simulink model "surgicalControl_Shared_memory_loop_2016b"  (R2016b)
settings: Solver=FixedStepAuto  StartTime=0.0  StopTime=inf  FixedStep=1/100  RelTol=1e-3
libraries: dspsigops x9, simulink x3, matlabGenericSHM_Block x1
settings Model: Creator=daniel  LastModifiedBy=crazy
settings OptimizationCC: LifeSpan=inf
settings DebuggingCC: SFExecutionAtInitializationDiag=none

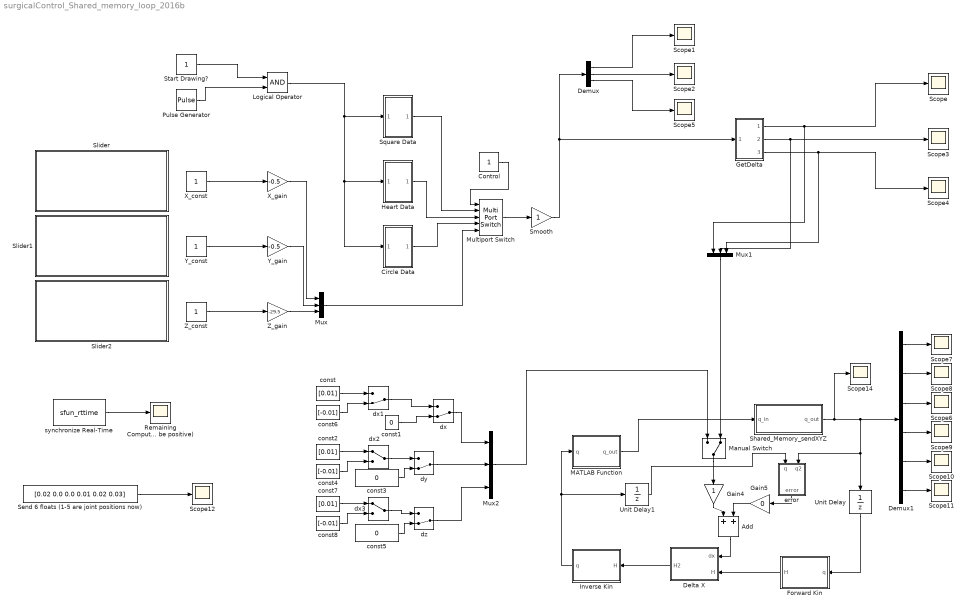
== system surgicalControl_Shared_memory_loop_2016b ==
  " GetDelta " : Subsystem
  " X_const " : Constant
  " Y_const" : Constant
  " Z_const" : Constant
  Add : Sum
  Circle Data : Subsystem
  "Control " : Constant
  Delta X : MATLAB Function  TreatAsAtomicUnit=on
  Demux : Demux  Outputs=3
  Demux1 : Demux  Outputs=6
  Forward Kin : MATLAB Function  TreatAsAtomicUnit=on
  Gain4 : Gain
  Gain5 : Gain  Gain=0
  Heart Data : Subsystem
  Inverse Kin : MATLAB Function  TreatAsAtomicUnit=on
  Logical Operator : Logic  AllPortsSameDT=off  OutDataTypeStr=boolean
  MATLAB Function : MATLAB Function  TreatAsAtomicUnit=on
  Manual Switch : ManualSwitch  CurrentSetting=0
  Multiport Switch : MultiPortSwitch  Inputs=4
  Mux : Mux  Inputs=3
  Mux1 : Mux  Inputs=3
  Mux2 : Mux  Inputs=3
  Pulse Generator : DiscretePulseGenerator  PulseType=Time based  Period=1  PulseWidth=20
  Remaining Computation Time (must be positive) : Scope
  Scope{,1..12,14} (14 alike) : Scope
  Send 6 floats (1-5 are joint positions now) : Constant  Value=[0.02 0.0 0.0 0.01 0.02 0.03]  OutDataTypeStr=single
  Shared_Memory_sendXYZ : Subsystem  mask{ID1=4}
  Slider : Subsystem  DialogController=hmiCreateDDGDialog  IsWebBlock=on  mask(MWDashboardBlock){webBlockId=4f94596f-dd6d-4e5e-bddc-7a8d913927f9, webBlockType=slider, ShowInLibBrowser=on, ShowInitialText=on, HMISrcModelName=surgicalControl_Shared_memory_loop_2016b}
      mask prompts: webBlockId "WebBlock Id"; webBlockType "WebBlock Type"; HMISrcModelName "Source Model"
      mask help: SimulinkHMI:dialogs:SliderDialogDesc
      mask Help: helpview([docroot '/mapfiles/simulink.map'], 'hmi_slider')
      mask Display:
      | if strcmp(get_param(bdroot(gcb),'BlockDiagramType'), 'library')
      |     image([(matlabroot) '/toolbox/simulink/hmi/icons/Slider.png']);
      | end
  Slider1 : Subsystem  DialogController=hmiCreateDDGDialog  IsWebBlock=on  mask(MWDashboardBlock){webBlockId=8aa996ad-7cd4-40fc-9a04-6a85939aea5d, webBlockType=slider, ShowInLibBrowser=on, ShowInitialText=on, HMISrcModelName=surgicalControl_Shared_memory_loop_2016b}
      mask prompts: webBlockId "WebBlock Id"; webBlockType "WebBlock Type"; HMISrcModelName "Source Model"
      mask help: SimulinkHMI:dialogs:SliderDialogDesc
      mask Help: helpview([docroot '/mapfiles/simulink.map'], 'hmi_slider')
      mask Display:
      | if strcmp(get_param(bdroot(gcb),'BlockDiagramType'), 'library')
      |     image([(matlabroot) '/toolbox/simulink/hmi/icons/Slider.png']);
      | end
  Slider2 : Subsystem  DialogController=hmiCreateDDGDialog  IsWebBlock=on  mask(MWDashboardBlock){webBlockId=1ddf6fd9-0225-4881-82ca-a25e179e2ab9, webBlockType=slider, ShowInLibBrowser=on, ShowInitialText=on, HMISrcModelName=surgicalControl_Shared_memory_loop_2016b}
      mask prompts: webBlockId "WebBlock Id"; webBlockType "WebBlock Type"; HMISrcModelName "Source Model"
      mask help: SimulinkHMI:dialogs:SliderDialogDesc
      mask Help: helpview([docroot '/mapfiles/simulink.map'], 'hmi_slider')
      mask Display:
      | if strcmp(get_param(bdroot(gcb),'BlockDiagramType'), 'library')
      |     image([(matlabroot) '/toolbox/simulink/hmi/icons/Slider.png']);
      | end
  Smooth : Gain
  "Square Data " : Subsystem
  Start Drawing? : Constant  SampleTime=1
  Unit Delay : UnitDelay  SampleTime=-1
  Unit Delay1 : UnitDelay  SampleTime=-1
  "X_gain " : Gain  Gain=-0.5
  "Y_gain " : Gain  Gain=-0.5
  Z_gain : Gain  Gain=-29.5
  const : Constant  Value=[0.01]  OutDataTypeStr=single
  const1 : Constant  Value=0  OutDataTypeStr=single
  const2 : Constant  Value=[0.01]  OutDataTypeStr=single
  const3 : Constant  Value=0  OutDataTypeStr=single
  const4 : Constant  Value=[-0.01]  OutDataTypeStr=single
  const5 : Constant  Value=0  OutDataTypeStr=single
  const6 : Constant  Value=[-0.01]  OutDataTypeStr=single
  const7 : Constant  Value=[0.01]  OutDataTypeStr=single
  const8 : Constant  Value=[-0.01]  OutDataTypeStr=single
  dx : ManualSwitch  CurrentSetting=0
  dx1 : ManualSwitch  CurrentSetting=0
  dx2 : ManualSwitch
  dx3 : ManualSwitch
  dy : ManualSwitch  CurrentSetting=0
  dz : ManualSwitch  CurrentSetting=0
  error : MATLAB Function  TreatAsAtomicUnit=on
  synchronize Real-Time : S-Function  FunctionName=sfun_rttime  Parameters=1  SFunctionDeploymentMode=off  EnableBusSupport=off
  wires:
  " GetDelta "/1(Out1) -> Mux1/1, Scope/1
  " GetDelta "/2(Out2) -> Scope3/1, Mux1/2
  " GetDelta "/3(Out3) -> Scope4/1, Mux1/3
  Multiport Switch/1 -> Smooth/1
  "Square Data "/1(xyz) -> Multiport Switch/2
  "Control "/1 -> Multiport Switch/1
  " X_const "/1 -> "X_gain "/1
  " Y_const"/1 -> "Y_gain "/1
  " Z_const"/1 -> Z_gain/1
  "X_gain "/1 -> Mux/1
  "Y_gain "/1 -> Mux/2
  Z_gain/1 -> Mux/3
  Mux/1 -> Multiport Switch/5
  Demux/2 -> Scope2/1
  Demux/1 -> Scope1/1
  Demux/3 -> Scope5/1
  synchronize Real-Time/1 -> Remaining Computation Time (must be positive)/1
  Smooth/1 -> Demux/1, " GetDelta "/1(In1)
  Shared_Memory_sendXYZ/1(q_out) -> Scope14/1, error/2(q2), Unit Delay/1, Demux1/1
  Demux1/3 -> Scope6/1
  Demux1/1 -> Scope7/1
  Demux1/2 -> Scope8/1
  Demux1/4 -> Scope9/1
  Demux1/5 -> Scope10/1
  Demux1/6 -> Scope11/1
  Send 6 floats (1-5 are joint positions now)/1 -> Scope12/1
  Forward Kin/1(H) -> Delta X/2(H)
  Delta X/1(H2) -> Inverse Kin/1(H)
  Unit Delay/1 -> Forward Kin/1(q)
  Mux1/1 -> Manual Switch/2
  Add/1 -> Delta X/1(dx)
  Mux2/1 -> Manual Switch/1
  dx/1 -> Mux2/1
  dx2/1 -> dy/1
  dy/1 -> Mux2/2
  dx3/1 -> dz/1
  dz/1 -> Mux2/3
  const/1 -> dx1/1
  const6/1 -> dx1/2
  const2/1 -> dx2/1
  const4/1 -> dx2/2
  const7/1 -> dx3/1
  const8/1 -> dx3/2
  const1/1 -> dx/2
  dx1/1 -> dx/1
  const3/1 -> dy/2
  const5/1 -> dz/2
  Inverse Kin/1(q) -> Unit Delay1/1, MATLAB Function/1(q)
  MATLAB Function/1(q_out) -> Shared_Memory_sendXYZ/1(q_in)
  Gain4/1 -> Add/1
  Manual Switch/1 -> Gain4/1
  error/1(error) -> Gain5/1
  Gain5/1 -> Add/2
  Unit Delay1/1 -> error/1(q)
  Pulse Generator/1 -> Logical Operator/2
  Start Drawing?/1 -> Logical Operator/1
  Logical Operator/1 -> Heart Data/1(In1), Circle Data/1(In1), "Square Data "/1(In1)
  Heart Data/1(xyz) -> Multiport Switch/3
  Circle Data/1(xyz) -> Multiport Switch/4

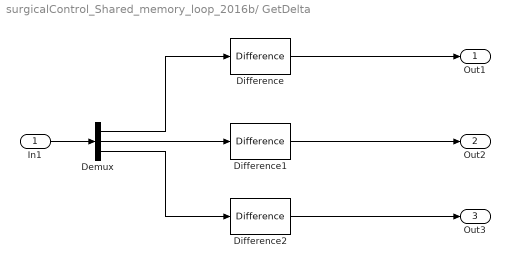
== system surgicalControl_Shared_memory_loop_2016b/ GetDelta  ==
  In1 : Inport
  Demux : Demux  Outputs=3
  Difference : simulink/Discrete/Difference  ICPrevInput=0  OutMin=[]  OutMax=[]  OutDataType=fixdt(1, 16)  OutScaling=2^-10  DoSatur=off
  Difference1 : simulink/Discrete/Difference  ICPrevInput=0  OutMin=[]  OutMax=[]  OutDataType=fixdt(1, 16)  OutScaling=2^-10  DoSatur=off
  Difference2 : simulink/Discrete/Difference  ICPrevInput=0  OutMin=[]  OutMax=[]  OutDataType=fixdt(1, 16)  OutScaling=2^-10  DoSatur=off
  Out1 : Outport
  Out2 : Outport  Port=2
  Out3 : Outport  Port=3
  wires:
  Difference1/1 -> Out2/1
  Difference/1 -> Out1/1
  Difference2/1 -> Out3/1
  In1/1 -> Demux/1
  Demux/1 -> Difference/1
  Demux/2 -> Difference1/1
  Demux/3 -> Difference2/1

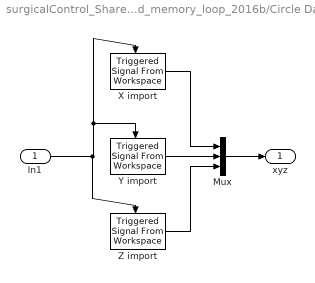
== system surgicalControl_Shared_memory_loop_2016b/Circle Data ==
  In1 : Inport
  Mux : Mux  Inputs=3
  X import : dspsigops/Triggered Signal From Workspace  Signal=xs_circle  TriggerType=Falling edge  ic=0  SamplesPerFrame=1  OutputAfterFinalValue=Setting to zero  OutputFrames=off
  Y import : dspsigops/Triggered Signal From Workspace  Signal=ys_circle  TriggerType=Falling edge  ic=0  SamplesPerFrame=1  OutputAfterFinalValue=Setting to zero  OutputFrames=off
  Z import : dspsigops/Triggered Signal From Workspace  Signal=zs_circle  TriggerType=Falling edge  ic=0  SamplesPerFrame=1  OutputAfterFinalValue=Setting to zero  OutputFrames=off
  xyz : Outport
  wires:
  X import/1 -> Mux/1
  Z import/1 -> Mux/3
  Mux/1 -> xyz/1
  Y import/1 -> Mux/2
  In1/1 -> Z import/Trigger, X import/Trigger, Y import/Trigger

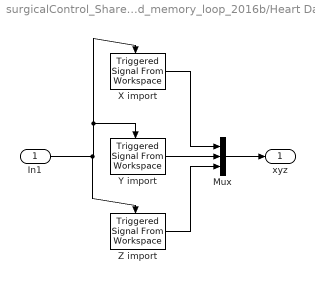
== system surgicalControl_Shared_memory_loop_2016b/Heart Data ==
  In1 : Inport
  Mux : Mux  Inputs=3
  X import : dspsigops/Triggered Signal From Workspace  Signal=xs_heart  TriggerType=Falling edge  ic=0  SamplesPerFrame=1  OutputAfterFinalValue=Setting to zero  OutputFrames=off
  Y import : dspsigops/Triggered Signal From Workspace  Signal=ys_heart  TriggerType=Falling edge  ic=0  SamplesPerFrame=1  OutputAfterFinalValue=Setting to zero  OutputFrames=off
  Z import : dspsigops/Triggered Signal From Workspace  Signal=zs_heart  TriggerType=Falling edge  ic=0  SamplesPerFrame=1  OutputAfterFinalValue=Setting to zero  OutputFrames=off
  xyz : Outport
  wires:
  X import/1 -> Mux/1
  Z import/1 -> Mux/3
  Mux/1 -> xyz/1
  Y import/1 -> Mux/2
  In1/1 -> Z import/Trigger, X import/Trigger, Y import/Trigger

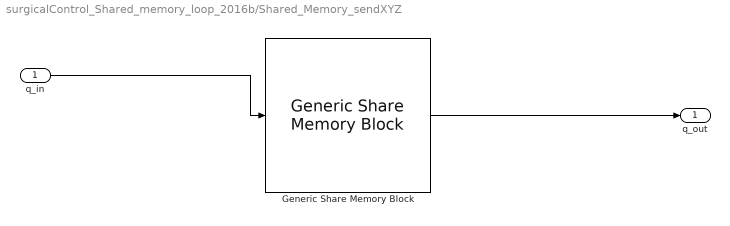
== system surgicalControl_Shared_memory_loop_2016b/Shared_Memory_sendXYZ ==
  q_in : Inport
  Generic Share Memory Block : matlabGenericSHM_Block/Generic Share Memory Block  nombre='EyeRob'  dispositivo=ID1  vecE=[6]  vecS=[6]  tipoE=['f']  tipoS=['f']
  q_out : Outport
  wires:
  q_in/1 -> Generic Share Memory Block/1
  Generic Share Memory Block/1 -> q_out/1

== system surgicalControl_Shared_memory_loop_2016b/Slider ==

== system surgicalControl_Shared_memory_loop_2016b/Slider1 ==

== system surgicalControl_Shared_memory_loop_2016b/Slider2 ==

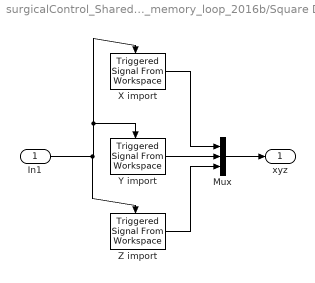
== system surgicalControl_Shared_memory_loop_2016b/Square Data  ==
  In1 : Inport
  Mux : Mux  Inputs=3
  X import : dspsigops/Triggered Signal From Workspace  Signal=xs_square  TriggerType=Falling edge  ic=0  SamplesPerFrame=1  OutputAfterFinalValue=Setting to zero  OutputFrames=off
  Y import : dspsigops/Triggered Signal From Workspace  Signal=ys_square  TriggerType=Falling edge  ic=0  SamplesPerFrame=1  OutputAfterFinalValue=Setting to zero  OutputFrames=off
  Z import : dspsigops/Triggered Signal From Workspace  Signal=zs_square  TriggerType=Falling edge  ic=0  SamplesPerFrame=1  OutputAfterFinalValue=Setting to zero  OutputFrames=off
  xyz : Outport
  wires:
  X import/1 -> Mux/1
  Z import/1 -> Mux/3
  Mux/1 -> xyz/1
  Y import/1 -> Mux/2
  In1/1 -> Z import/Trigger, X import/Trigger, Y import/Trigger

== matlab function surgicalControl_Shared_memory_loop_2016b/Inverse Kin ==
  data: H input; q output
function q = fcn(H)

q = IK(H)';

== matlab function surgicalControl_Shared_memory_loop_2016b/Forward Kin ==
  data: q input; H output
function H = fcn(q)
H = fKin(q');

== matlab function surgicalControl_Shared_memory_loop_2016b/Delta X ==
  data: dx input; H input; H2 output
function H2 = fcn(dx,H)
H2 = H;
H2(1,4)=H2(1,4)+dx(3,1);
H2(2,4)=H2(2,4)+dx(2,1);
H2(3,4)=H2(3,4)+dx(1,1);
end

== matlab function surgicalControl_Shared_memory_loop_2016b/error ==
  data: q input; error output; q2 input
function error = fcn(q,q2)
H1 = fKin(q');
H2 = fKin(q2');
H=H1-H2;
error=H(1:3,4)';
end

== matlab function surgicalControl_Shared_memory_loop_2016b/MATLAB Function ==
  data: q input size=[1 6]; q_out output size=[1 6]
function q_out = correctForPrismatic(q)
%#codegen
 if iscolumn(q)
       q = q';
 end
q_out=zeros(1, 6,'single');

q1=q(1,1);
q2=q(1,2);
q3=q(1,3);
q4=q(1,4);
q2_temp= getL2(q1,q2);
q4_temp= getL1(q3,q4);

% end


q_out(1,1) = q1;
q_out(1,2) = q2_temp;
q_out(1,3) = q3;
q_out(1,4) = q4_temp;
q_out(1,5) = q(1,5);
q_out(1,6) = q(1,6);
end
